simulink model "CorneringStiffness"  (R2024b)
settings: Solver=VariableStepAuto  StartTime=0  StopTime=30  RelTol=1e-3
libraries: simulink x6
settings Model: Creator=owen  LastModifiedBy=owen

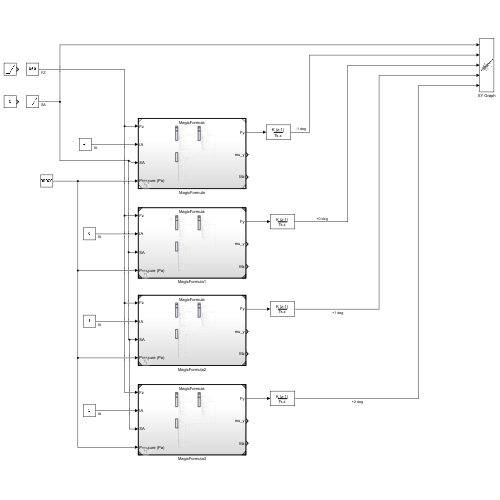
[thumbnail: Simulink's stored preview of the top-level diagram]
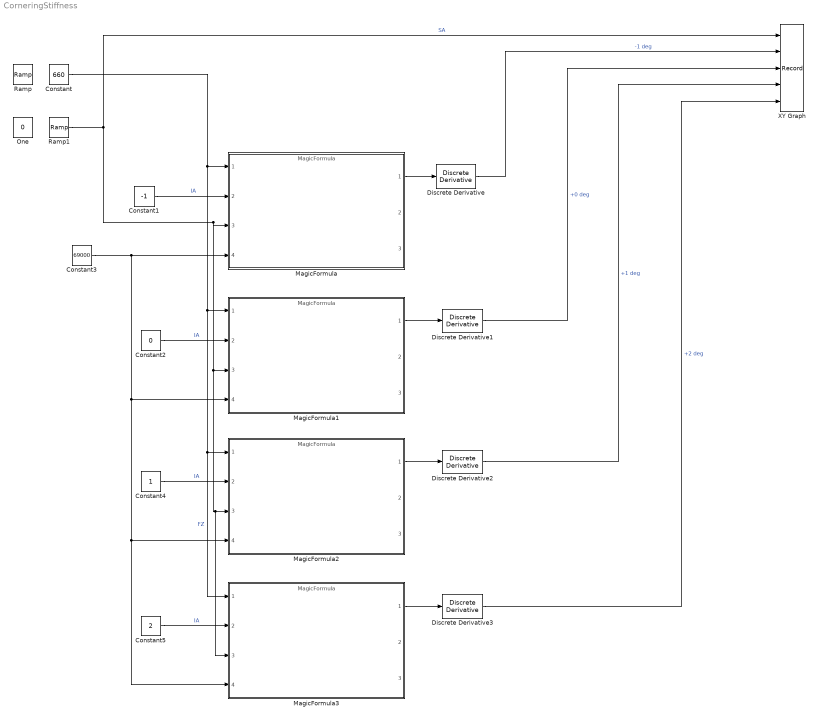
== system CorneringStiffness ==
  Constant : Constant  Value=660
  Constant1 : Constant  Value=-1
  Constant2 : Constant  Value=0
  Constant3 : Constant  Value=69000
  Constant4 : Constant
  Constant5 : Constant  Value=2
  Discrete Derivative{,1..3} (4 alike) : simulink/Discrete/Discrete Derivative  gainval=-1  ICPrevScaledInput=0.0  OutMin=[]  OutMax=[]  OutDataType=fixdt(1, 16)  OutScaling=2^-10  DoSatur=off
  MagicFormula{,1..3} (4 alike) : ModelReference  ModelNameDialog=MagicFormula.slx  SimulationMode=Normal  ModelReferenceVersion=1.53
  One : Constant  Value=0  OutDataTypeStr=Inherit: Inherit via back propagation
  Ramp : simulink/Sources/Ramp  slope=1  start=0  InitialOutput=0
  Ramp1 : simulink/Sources/Ramp  slope=1  start=0  InitialOutput=-15
  XY Graph : Record  FileSettingsInternal="{\"entries\":[{\"content\":{\"excelSettings\":{\"content\":{},\"type\":\"Streamout.ExcelSettings\"}},\"type\":\"Streamout.FileSettingStorage\",\"uuid\":\"\"}],\"packageUris\":[\"http:\\/\\/schema.mathworks.com\\/mf0\\/streamout_blocks\\/R2020a\"],\"version\":\"1.0\"}"  Layout=[1 1]  SignalsInternal="{\"entries\":[{\"content\":{\"signals\":[{\"content\":{\"blockPath\":[],\"dimensions\":[1],\"domain\":\"\",\"lineColor\":\"#fe330a\",\"lineWidth\":2,\"port\":1,\"sid\":[\"\"],\"signalID\":1,\"signalName\":\"SA\"},\"type\":\"RecordBlkView.Signal\",\"uuid\":\"\"},{\"content\":{\"blockPath\":[],\"dimensions\":[1],\"domain\":\"\",\"lineColor\":\"#22b573\",\"lineWidth\":2,\"port\":2,\"sid\":[\"\"],\"signalID\":2,\"signalName\":\"-1 deg\"},\"type\":\"RecordBlkView.Signal\",\"uuid\":\"\"},{\"content\":{\"blockPath\":[],\"dimensions\":[1],\"domain\":\"\",\"lineColor\":\"#0072bd\",\"lineWidth\":2,\"port\":3,\"sid\":[\"\"],\"signalID\":3,\"signalName\":\"+0 deg\"},\"type\":\"RecordBlkView.Signal\",\"uuid\":\"\"},{\"content\":{\"blockPath\":[],\"dimensions\":[1],\"domain\":\"\",\"lineColor\":\"#d95319\",\"lineWidth\":2,\"port\":4,\"sid\":[\"\"],\"signalID\":4,\"signalName\":\"+1 deg\"},\"type\":\"RecordBlkView.Signal\",\"uuid\":\"\"},{\"content\":{\"blockPath\":[],\"dimensions\":[1],\"domain\":\"\",\"lineColor\":\"#edb120\",\"lineWidth\":2,\"port\":5,\"sid\":[\"\"],\"signalID\":5,\"signalName\":\"+2 deg\"},\"type\":\"RecordBlkView.Signal\",\"uuid\":\"\"}]},\"type\":\"RecordBlkView.InputSignals\",\"uuid\":\"\"}],\"packageUris\":[\"http:\\/\\/schema.mathworks.com\\/mf0\\/streamout_blocks\\/R2020a\"],\"version\":\"1.0\"}"  VisualizationBindings="{\"xyplotplugin\":{\"info\":[{\"series\":[],\"subplotID\":1}]}}"  CompatibilityTag=XY
  wires:
  Constant/1 -> MagicFormula3/1, MagicFormula2/1, MagicFormula1/1, MagicFormula/1  "FZ"
  Ramp1/1 -> XY Graph/1, MagicFormula3/3, MagicFormula2/3, MagicFormula1/3, MagicFormula/3  "SA"
  Constant1/1 -> MagicFormula/2  "IA"
  Discrete Derivative/1 -> XY Graph/2  "-1 deg"
  Constant3/1 -> MagicFormula3/4, MagicFormula2/4, MagicFormula1/4, MagicFormula/4
  Discrete Derivative3/1 -> XY Graph/5  "+2 deg"
  Discrete Derivative2/1 -> XY Graph/4  "+1 deg"
  Discrete Derivative1/1 -> XY Graph/3  "+0 deg"
  MagicFormula/1 -> Discrete Derivative/1
  MagicFormula1/1 -> Discrete Derivative1/1
  MagicFormula2/1 -> Discrete Derivative2/1
  MagicFormula3/1 -> Discrete Derivative3/1
  Constant2/1 -> MagicFormula1/2  "IA"
  Constant4/1 -> MagicFormula2/2  "IA"
  Constant5/1 -> MagicFormula3/2  "IA"
